simulink model "visualservoingomni"  (Simulink 5.0)
settings: Solver=ode45  StartTime=0.0  StopTime=35.0  RelTol=1e-3
libraries: simulink x1
settings Model: LastModifiedBy=hoffmann  BooleanDataType=off

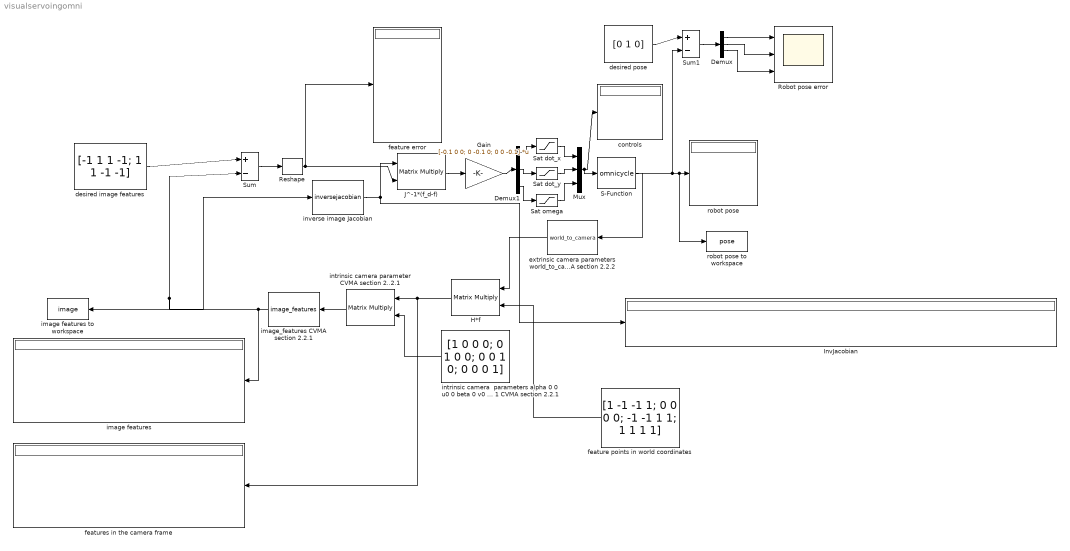
== system visualservoingomni ==
  Demux : Demux  Outputs=3
  Demux1 : Demux  Outputs=3
  Gain : Gain  Gain=[-0.1 0 0; 0 -0.1 0; 0 0 -0.1]  Multiplication=Matrix(K*u)  SaturateOnIntegerOverflow=on
  H*f : Product  Orientation=left  Multiplication=Matrix(*)  SaturateOnIntegerOverflow=on
  InvJacobian : Display
  J^-1*(f_d-f) : Product  Multiplication=Matrix(*)  SaturateOnIntegerOverflow=on
  Mux : Mux  Inputs=3
  Reshape : simulink/Math Operations/Reshape  OutputDimensionality=1-D array  OutputDimensions=[1,1]
  Robot pose error : Scope  NumInputPorts=3
      settings: YMin=-5~-5~-5  YMax=5~5~5
  S-Function : S-Function  FunctionName=omnicycle
  Sat dot_x : Saturate
  Sat dot_y : Saturate
  Sat omega : Saturate  UpperLimit=0.1  LowerLimit=-0.1
  Sum : Sum  Inputs=|+-  SaturateOnIntegerOverflow=on
  Sum1 : Sum  Inputs=|+-  SaturateOnIntegerOverflow=on
  "controls " : Display
  desired image features : Constant  Value=[-1 1 1 -1; 1 1 -1 -1]
  desired pose : Constant  Value=[0 1 0]
  extrinsic camera parameters world_to_camera cos theta sin theta 0 -x cos theta - y sin theta -sin theta cos theta 0 -y cos theta +x sin theta 0 0 1 z 0 0 0 1 CVMA section 2.2.2 : MATLABFcn  Orientation=left  MATLABFcn=world_to_camera  OutputDimensions=[4 4]  OutputSignalType=real  Output1D=off
  feature error : Display
  feature points in world coordinates : Constant  Orientation=left  Value=[1 -1 -1 1; 0 0 0 0; -1 -1 1 1; 1 1 1 1]
  features in the camera frame : Display
  image features : Display
  image features to workspace : ToWorkspace  VariableName=image  SampleTime=0.1  SaveFormat=Array
  image_features CVMA section 2.2.1 : MATLABFcn  Orientation=left  MATLABFcn=image_features  OutputSignalType=real  Output1D=off
  "intrinsic camera parameter CVMA section 2..2.1 " : Product  Orientation=left  Multiplication=Matrix(*)  SaturateOnIntegerOverflow=on
  "intrinsic camera  parameters alpha 0 0 u0 0 beta 0 v0 0 0 1 0 0 0 0 1 CVMA section 2.2.1  " : Constant  Orientation=left  Value="[1 0 0 0; 0 1 0 0;  0 0 1 0; 0 0 0 1]"  VectorParams1D=off
  inverse image Jacobian : MATLABFcn  MATLABFcn=inversejacobian  OutputDimensions=[3 8]  OutputSignalType=real  Output1D=off
  robot pose : Display
  robot pose to workspace : ToWorkspace  VariableName=pose  SampleTime=0.1  SaveFormat=Array
  wires:
  S-Function/1 -> extrinsic camera parameters world_to_camera cos theta sin theta 0 -x cos theta - y sin theta -sin theta cos theta 0 -y cos theta +x sin theta 0 0 1 z 0 0 0 1 CVMA section 2.2.2/1, Sum1/2, robot pose/1, robot pose to workspace/1
  extrinsic camera parameters world_to_camera cos theta sin theta 0 -x cos theta - y sin theta -sin theta cos theta 0 -y cos theta +x sin theta 0 0 1 z 0 0 0 1 CVMA section 2.2.2/1 -> H*f/1
  feature points in world coordinates/1 -> H*f/2
  H*f/1 -> features in the camera frame/1, "intrinsic camera parameter CVMA section 2..2.1 "/1
  image_features CVMA section 2.2.1/1 -> image features/1, Sum/2, inverse image Jacobian/1, image features to workspace/1
  desired image features/1 -> Sum/1
  inverse image Jacobian/1 -> J^-1*(f_d-f)/1, InvJacobian/1
  Sum/1 -> Reshape/1
  Reshape/1 -> J^-1*(f_d-f)/2, feature error/1
  J^-1*(f_d-f)/1 -> Gain/1
  Demux/1 -> Robot pose error/1
  Demux/2 -> Robot pose error/2
  Demux/3 -> Robot pose error/3
  desired pose/1 -> Sum1/1
  Sum1/1 -> Demux/1
  Gain/1 -> Demux1/1
  Mux/1 -> S-Function/1, "controls "/1
  Demux1/1 -> Sat dot_x/1
  Sat dot_x/1 -> Mux/1
  Demux1/2 -> Sat dot_y/1
  Sat dot_y/1 -> Mux/2
  Demux1/3 -> Sat omega/1
  Sat omega/1 -> Mux/3
  ? -> ?
  "intrinsic camera parameter CVMA section 2..2.1 "/1 -> image_features CVMA section 2.2.1/1
  "intrinsic camera  parameters alpha 0 0 u0 0 beta 0 v0 0 0 1 0 0 0 0 1 CVMA section 2.2.1  "/1 -> "intrinsic camera parameter CVMA section 2..2.1 "/2
